simulink model "LongLatDriveline"  (R2024b)
settings: Solver=FixedStepAuto  StartTime=0  StopTime=120  FixedStep=0.002  RelTol=1e-3
InitFcn:
  | load('waypoints.mat');
  | VehicleObj = Simulink.data.dictionary.open('./ModelData/VehicleData.sldd');
  | %dDataSectObj = getSection(myDictionaryObj,'Design Data');
StopFcn:
  | Plot_LateralModelErrorControl;
  | 
  | mdlWks = get_param(gcs, 'ModelWorkspace');
  | par_ToDrvDesigner = evalin(mdlWks, 'ToDrvDesigner');
  | 
  | if par_ToDrvDesigner.Value
  |     ExportdrivingScenario;
  | end
model workspace (MAT data in the model file):
  ToDrvDesigner : Simulink.Parameter (value not decoded)
values from neighbouring files (symbols this model uses):
  A_F = 2.341157    [VehicleData.sldd]
  C_af = 80000.0    [VehicleData.sldd]
  C_ar = 80000.0    [VehicleData.sldd]
  C_d = 0.24    [VehicleData.sldd]
  f = 0.01    [VehicleData.sldd]
  g = 9.81    [VehicleData.sldd]
  h_aero = 0.65    [VehicleData.sldd]
  h_gc = 0.65    [VehicleData.sldd]
  Iz = 2873.0    [VehicleData.sldd]
  lf = 1.1    [VehicleData.sldd]
  lr = 1.58    [VehicleData.sldd]
  m = 2238.932    [VehicleData.sldd]
  Nf = 2.0    [VehicleData.sldd]
  Nr = 2.0    [VehicleData.sldd]
  r_stat = 0.342    [VehicleData.sldd]
  r_w = 0.352    [VehicleData.sldd]
  rho = 1.225    [VehicleData.sldd]
  theta = 0.0    [VehicleData.sldd]
  transGear = 0.1027    [VehicleData.sldd]
  V_wind = 0.0    [VehicleData.sldd]
symbols that are objects in the model workspace (value not decoded): ToDrvDesigner
undefined symbols (not defined in the file or in its folder): InitialPsi, InitialX, InitialY, phi
libraries: slpidlib x14, spsMosfetLib x6, simulink x4, spsVoltageMeasurementLib x3, SignalEditorBlockLib x2, spsDCVoltageSourceLib x1, spspowerguiLib x1
(part 5 of 5)

== matlab function LongLatDriveline/GetRefference ==
  data: e1 output size=1; de1 output; e2 output; de2 output; e3 output; Vx_reff output; dPsi_des output; X input size=1; Y input double size=1; racetrackwaypoints parameter; Psi input; dPsi input; Vy input; Vx input; phi_ref output
% ******************* GetRefference *********************
%*********************************************************************
% Author: L.Arturo Torres-Romero
% Date: 22-10-2020
% BICYCLE MODEL OF LATERAL VEHICLE DYNAMICS
% Based on Rajamani chapter 2.3 page 30 and  in the next publication with
% the controller
% https://www.researchgate.net/publication/340166902_LATERAL_VEHICLE_DYNAMICS_AND_CONTROLLERS_DESIGN
% This block gets the errors required for the controller of the steering wheel that is based in the error respect the road.
% In this case the road is specified as a list of points (waypoints) in the array racetrackwaypoints
%******************************************************************
%******************* INPUTS DESCRIPTIONS **************************
%******************************************************************
% X:   Global coordinate X of the C.G. of the vehicle 
% Y:   Global coordinate X of the C.G. of the vehicle
% racetrackwaypoints: array with a list of waypoints of the road [X Y]
% Psi: Is the yaw angle respect to the inertial global system
% dPsi: Angular velocity of the yaw angle.
% Vy: Lateral velocity
% Vx: Longitudinal velocity
%******************************************************************
% ******************* OUTPUTS DESCRIPTIONS ************************
%******************************************************************
% e1  : is the lateral position error respect the road.
% de1 : derivative of e1.
% e2  : is the yaw angle error with respect the road. 
% de2 : derivarive of the e2.
% e3  :
% Vx  :
% Vx_reff  : Longitudinal speed from the waypoints.
% dPsi_des : Yaw derivative according the actual speed and road.
% phi_ref  : Superelevation of the road defined in the waipoints file

function [e1,de1,e2,de2,e3,Vx_reff,dPsi_des,phi_ref] = GetReff(X,Y,racetrackwaypoints, Psi,dPsi, Vy, Vx) 
% functions declared as extrinsic to avoid code generator try to generate
% code from them
coder.extrinsic('msgbox');
coder.extrinsic('set_param');
coder.extrinsic('uiwait');
coder.extrinsic('movegui');
coder.extrinsic('imread');
%-----------------------------

persistent lastK;
if isempty(lastK) % initialization of lastK
    lastK = int32(1); 
end

PQ = [X,Y]; % current Intertial position of vehicle
P = racetrackwaypoints(lastK:end,1:2); % List of waypoints column1 = X coord.  column2 = Y coord. Column 3 = Vx for reference
[k,D] = knnsearch_lib(P,PQ,1); % locate the closest waypoint to the vehicle. k = index, D = distance
k = k(1);

% this is to avoid searching in waypoints already behind the vehicle.
if k > lastK % if we are ahead of the last point searched, then discard the points behind.
    lastK = k-1;
end

% here we take 3 points: the closest, one behind, one in front.
P_road1 = P(k-1,:);
P_road2 = P(k,:);
P_road3 = P(k+1,:);
Vx_reff = racetrackwaypoints(k,3);
Vx_reff = Vx_reff(1);

LookAhead = 5; %how many points ahead to look for the orientation error

if k+LookAhead >= size(P,1)-1 % condition to stop simmulation
    % Display a message dialog

    [img, map] = imread('images/EndFlag.png'); % Cargar la imagen
    h = msgbox('You have arrived!!!', 'Simulation Stop', 'custom', img, map);
    movegui(h, 'northwest');
    % Stop the simulation
    set_param(bdroot, 'SimulationCommand', 'stop');
end

F = atan2( (P(k+LookAhead,2)-P(k,2)),(P(k+LookAhead,1)-P(k,1))); % Obtaining the road orientation
psi_des = F(1);
psi_des = wrapTo2Pi(psi_des);

P_veh = PQ - P_road2;

% Convert from intertial coordinates system to body fixed system. C.G. as
% center and rotated Psi degrees.
M_Rot = [cos(psi_des) -sin(psi_des); sin(psi_des) cos(psi_des)];
P_veh = P_veh*M_Rot;

e1 = P_veh(2); % error e1 that is the y distance from C.G. to desired waypoint from the vehicle reference.
e2 = Psi - psi_des; % error e2 which is the error in the orientation.
e2 = mod(e2 + pi, 2*pi) - pi; % angle adjusted and bounded to -pi to pi.

de1 = Vy + Vx*(e2); % derivative of e1

e3 = P_veh(1); % error e1 that is the x distance from C.G. to desired waypoint from the vehicle reference.

% Obtainig the radius of imaginary circle of the curve
Xc = [P_road1(1);P_road2(1);P_road3(1)];
Yc = [P_road1(2);P_road2(2);P_road3(2)];
[xc,yc,R,a] = circfit(Xc,Yc);
C = [xc yc];
C = (C-P_road2)*M_Rot;
xc = C(1);
yc = C(2);
R = R*sign(yc);


%in streight line, the radius falls into singularity. here is detected
%and solved with a minimum
eval = ~isfinite(R);
if eval
 R = 100000; % in case of NaN define a straight line as an arc of circle of R very big.
end

dPsi_des = Vx/R; % derivative of orientation refference
de2 = dPsi - dPsi_des; % derivative of e2


% sueperelevation of the road or banking
phi_ref = atan(Vx^2/(127*R)); % change for Vx_ref when it is reaady

end

== matlab function LongLatDriveline/LateralController/HOSMC_IntegralBlocksSuperTwistingV2/HOSMC_SuperTwistingV2 ==
  data: U output size=1; dz output; dv0 output size=[2 1]; E input; Vx input; dPsi_des input; phi_ref input; z input; v0 input size=[2 1]; v1 input size=2; C_af parameter; g parameter; C_ar parameter; lf parameter; lr parameter; Iz parameter; m parameter; dv1 output size=[2 1]; d_0 output; d_1 output
% ******************* Lateral dynamic controller *********************

%*********************************************************************
% Author: L.Arturo Torres-Romero
% Date: 22-10-2025
% This controller controlls the direction of a car, based in the dynamics
% of the Block Controller with Integral Super-Twisting Algorithm.
% The main control, is a linear control by blocks. integral super-twisting
% SMC is used to eliminate disturbances.
% Torres-Romero, L.A.; González-Jiménez, L.E. A Block Controller with 
% Integral Super-Twisting Algorithm for the Path Following of a 
% Self-Driving Electric Vehicle Considering Actuator Dynamics. World 
% Electr. Veh. J. 2025, 16, 643. https://doi.org/10.3390/wevj16120643 
%******************* PARAMETERS DESCRIPTIONS **********************
%******************************************************************
% m: vehicle mass
% g: gravity
% C_af : Cornering  stiffness  of  front  wheels.
% C_ar : Cornering  stiffness  of  rear  wheels.
% lf : distance fron the center of gravity to the front wheel axis.
% lr : distance fron the center of gravity to the rear wheel axis.
% Iz : this is the momentum of inertia of the vehicle respect the z axis.
%******************************************************************
%******************* INPUTS DESCRIPTIONS **************************
%******************************************************************
% E:   (column vector)[e1;de1;e2;de2] states of the state space of 
%       the system that includes the errors as follows:
%      e1  : is the lateral position error respect the road.
%      de1 : derivative of e1.
%      e2  : is the yaw angle error with respect the road. 
%      de2 : derivarive of the e2.
% Vx: Logitudinal velocity.
% dPsi_des : Yaw derivative according the actual speed and road.
% phi_ref  : Superelevation of the road defined in the waipoints file
% z        : Integral part of the second block
% v0       : Switching control of the first Super-Twisting (Integrated)
% v1       : Switching control of the second Super-Twisting (Integrated)

%******************************************************************
% ******************* OUTPUTS DESCRIPTIONS ************************
%******************************************************************
% U: control coutput in radians. Angle of the frontal wheels respect to the
%    longitudinal axis
% dz  : Integral part of the second block (to be integrated)
% dv0 : Switching control of the first Super-Twisting
% dv1 : Switching control of the second Super-Twisting
% d_0 : Control of the first block.
% d_1 : Control of the second block.
%******************************************************************

function [U,dz,dv0,dv1, d_0,d_1] = HOSMC_SuperTwistingCtrl...
    (E, Vx,dPsi_des, phi_ref,z,v0,v1, C_af, g, C_ar, lf, lr, Iz, m) 
Y1 = [0;0];
Y2 = [0;0];

Y1 = [E(1);E(3)];
Y2 = [E(2);E(4)];

phi = phi_ref;

%**************************************************
%******* Matrix A formulation *********************
A211 = -(2*C_af + 2*C_ar)/(m*Vx);
A112 = (2*C_af + 2*C_ar)/m;
A212 = (-2*C_af*lf + 2*C_ar*lr)/(m*Vx);
A221 = -(2*C_af*lf - 2*C_ar*lr)/(Iz*Vx);
A122 = (2*C_af*lf - 2*C_ar*lr)/Iz;
A222 = -(2*C_af*lf^2 + 2*C_ar*lr^2)/(Iz*Vx);

A1 = [0 A112;0 A122];
A2 = [A211 A212;A221 A222];

%**************************************************
%******* Matrix B1 formulation ********************
B1_2 = 2*C_af/m;
B1_4 = 2*C_af*lf/Iz;

B1 = [B1_2;B1_4];
%***************************************************

%***************************************************
%******* Matrix L formulation *********************
l1 = (A212 - Vx)*dPsi_des +g*sin(phi);
l2 = A222*dPsi_des;
L = [l1;l2];

%***************************************************
%%
%%%%%%%%%%%%%% SUPER TWISTING 1 %%%%%%%%%%%%%%%%%
% %*********** Controller parameters **************
%***************************************
k1 =   6*[5 1  ;1 1  ];
ku0 =  1;
kv0 =  1;

ku1 =  1;
kv1 =  1;

e = -k1*Y1 -Y2;
s = e + z;

d_0 = -B1\(A1*Y1 + (k1*eye(2) + A2)*Y2 + L -ku0*sqrt(abs(e)).*sign(e) + v0);
dv0 = -kv0*sign(e);

d_1 = -B1\(-ku1*sqrt(abs(s)).*sign(s) + v1);
dv1 = -kv1*sign(s);

dz = A1*Y1 + (k1*eye(2) + A2)*Y2 + L + B1*d_0;

%***********************************************

%ctrlVal = d_0;
ctrlVal = d_0 + d_1;
U = real(ctrlVal);

== matlab function LongLatDriveline/SteerActuator/BLDC_AngleCtrl/ParkClarke ==
  data: X_abc input; Y_dq output; theta input
function Y_dq = fcn(X_abc, theta)

% Park clarke transform eliminating the third element
PC_T = (sqrt(2)/2)*[sqrt(3)*cos(theta)  sin(theta)  -sin(theta) ; ...
                    -sqrt(3)*sin(theta)  cos(theta)  -cos(theta)];

Y_dq =PC_T*X_abc;
end

== matlab function LongLatDriveline/LateralController/DirectLyapunov ==
  data: U output size=1; E input; Vx input; dPsi_des input; C_af parameter; g parameter; C_ar parameter; lf parameter; lr parameter; Iz parameter; m parameter
% ******************* Lateral dynamic controller *********************
%*********************************************************************
% Author: L.Arturo Torres-Romero
% Date: 22-10-2020
% This controller controlls the direction of a car, based in the dynamics
% described  in the next link and using the Direct Lyapunov formulation: 
% https://www.researchgate.net/publication/340166902_LATERAL_VEHICLE_DYNAMICS_AND_CONTROLLERS_DESIGN
%
%ALCALÁ, Eugenio, et al. Comparison of two non-linear model-based control strategies for autonomous vehicles. 
% En 2016 24th Mediterranean Conference on Control and Automation (MED). IEEE, 2016. p. 846-851.
%******************* PARAMETERS DESCRIPTIONS **********************
%******************************************************************
% m: vehicle mass
% g: gravity
% C_af : Cornering  stiffness  of  front  wheels.
% C_ar : Cornering  stiffness  of  rear  wheels.
% lf : distance fron the center of gravity to the front wheel axis.
% lr : distance fron the center of gravity to the rear wheel axis.
% Iz : this is the momentum of inertia of the vehicle respect the z axis.
%******************************************************************
%******************* INPUTS DESCRIPTIONS **************************
%******************************************************************
% E:   (column vector)[e1;de1;e2;de2] states of the state space of 
%       the system that includes the errors as follows:
%      e1  : is the lateral position error respect the road.
%      de1 : derivative of e1.
%      e2  : is the yaw angle error with respect the road. 
%      de2 : derivarive of the e2.
% Vx: Logitudinal velocity.

%******************************************************************
% ******************* OUTPUTS DESCRIPTIONS ************************
%******************************************************************
% U: control coutput in radians. Angle of the frontal wheels respect to the
%    longitudinal axis
% isCtrl: when true means that the matrix Mc has full rank, and hence, the
%         system is controllable
%******************************************************************

function U = DirectLyapunovCtrl(E, Vx,dPsi_des, C_af, g, C_ar, lf, lr, Iz, m) % pd polos deseados

psi_e = E(3);
y_e = E(1);
L = lf+lr;
k2 = 1.1;
k3 = 3;

dPsi_ctrl = dPsi_des -k2*Vx*(sin(psi_e)/psi_e)*y_e - k3*psi_e;

ctrlVal = atan((L*dPsi_ctrl)/Vx);


U = real(ctrlVal);
